simulink model "Desacople_RetroA_Fisica_Compensacion"  (R2023b)
settings: Solver=VariableStepAuto  StartTime=0.0  StopTime=10.0  RelTol=1e-3
values from neighbouring files (symbols this model uses):
  lambda_m = 0.016    [parametros_proyecto2.m]
undefined symbols (not defined in the file or in its folder): L_d, L_q, P_p
settings Model: Creator=ignab  LastModifiedBy=ignab

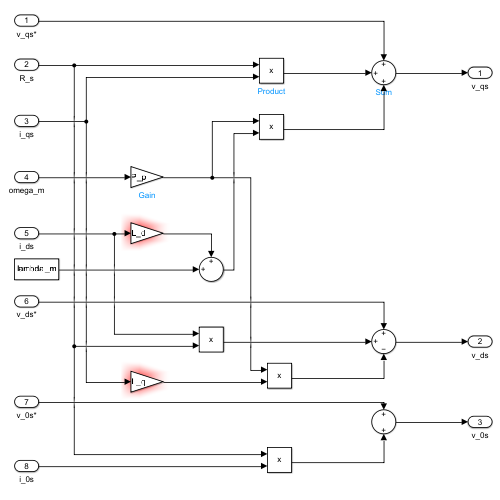
[thumbnail: Simulink's stored preview of the top-level diagram]
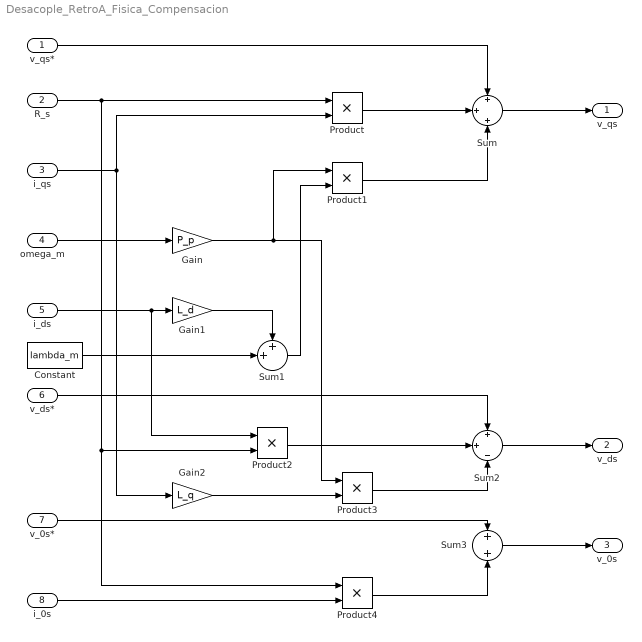
== system Desacople_RetroA_Fisica_Compensacion ==
  v_qs* : Inport
  R_s : Inport  Port=2
  i_qs : Inport  Port=3
  omega_m : Inport  Port=4
  i_ds : Inport  Port=5
  v_ds* : Inport  Port=6
  v_0s* : Inport  Port=7
  i_0s : Inport  Port=8
  Constant : Constant  Value=lambda_m
  Gain : Gain  Gain=P_p
  Gain1 : Gain  Gain=L_d
  Gain2 : Gain  Gain=L_q
  Product{,1..4} (5 alike) : Product
  Sum : Sum  Inputs=+|+|+
  Sum1 : Sum  Inputs=++|
  Sum2 : Sum  Inputs=+|+|-
  Sum3 : Sum  Inputs=+|+
  v_qs : Outport
  v_ds : Outport  Port=2
  v_0s : Outport  Port=3
  wires:
  R_s/1 -> Product4/1, Product2/2, Product/1
  Product/1 -> Sum/2
  v_qs*/1 -> Sum/1
  i_qs/1 -> Gain2/1, Product/2
  Product1/1 -> Sum/3
  Gain/1 -> Product3/1, Product1/1
  omega_m/1 -> Gain/1
  i_ds/1 -> Product2/1, Gain1/1
  Constant/1 -> Sum1/2
  Gain1/1 -> Sum1/1
  Sum1/1 -> Product1/2
  Sum/1 -> v_qs/1
  v_ds*/1 -> Sum2/1
  Gain2/1 -> Product3/2
  Product3/1 -> Sum2/3
  Product2/1 -> Sum2/2
  i_0s/1 -> Product4/2
  v_0s*/1 -> Sum3/1
  Product4/1 -> Sum3/2
  Sum3/1 -> v_0s/1
  Sum2/1 -> v_ds/1
